simulink model "test_Heaters_Simulink"  (R2016a)
settings: Solver=FixedStepAuto  StartTime=0.0  StopTime=inf  RelTol=1e-3
libraries: arduinolib x5, simulink x1
settings Model: SimulationMode=external  ExtModeTrigDuration=2  Creator=johnh  LastModifiedBy=johnh
settings OptimizationCC: OptimizeModelRefInitCode=on  LifeSpan=1  MaxStackSize=64
settings HardwareCC: ProdBitPerInt=16  ProdBitPerPointer=16  ProdLargestAtomicFloat=None  ProdWordSize=8  ProdHWDeviceType=Atmel->AVR  UseEmbeddedCoderFeatures=off  UseSimulinkCoderFeatures=off
settings RTWCC: SystemTargetFile=ert.tlc  HardwareBoard=Arduino Uno  TemplateMakefile=ert_default_tmf  GenerateReport=on  Toolchain=Arduino AVR v1.6.1  BuildConfiguration=Faster Runs  IncludeHyperlinkInReport=on  LaunchReport=on  GenerateTraceInfo=on  GenerateTraceReport=on  GenerateTraceReportSl=on  GenerateTraceReportSf=on  GenerateTraceReportEml=on
settings CodeAppCC: ForceParamTrailComments=on  IgnoreCustomStorageClasses=off  OperatorAnnotations=on  SimulinkDataObjDesc=on  SFDataObjDesc=on  MATLABFcnDesc=on  InsertBlockDesc=on  MATLABSourceComments=on
settings ERTTargetCC: SupportContinuousTime=on  SupportNonInlinedSFcns=on  SupportVariableSizeSignals=on

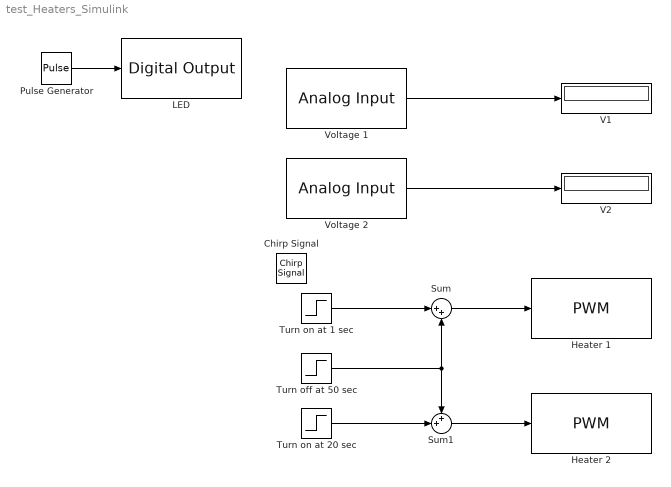
== system test_Heaters_Simulink ==
  Heater 1 : arduinolib/PWM  pinNumber=3  blockPlatform=arduino
  Heater 2 : arduinolib/PWM  pinNumber=5  blockPlatform=arduino
  LED : arduinolib/Digital Output  pinNumber=9  blockPlatform=arduino
  Pulse Generator : DiscretePulseGenerator  Period=10  PulseWidth=5  SampleTime=0.1
  Sum : Sum  Inputs=|++
  Sum1 : Sum  Inputs=++|
  Turn off at 50 sec : Step  Time=50  After=-100  SampleTime=0.1
  Turn on at 1 sec : Step  After=100  SampleTime=0.1
  Turn on at 20 sec : Step  Time=20  After=100  SampleTime=0.1
  V1 : Display
      settings: Decimation=3
  V2 : Display
      settings: Decimation=3
  Voltage 1 : arduinolib/Analog Input  pinNumber=0  sampleTime=0.1  blockPlatform=arduino
  Voltage 2 : arduinolib/Analog Input  pinNumber=2  sampleTime=0.1  blockPlatform=arduino
  Chirp Signal : simulink/Sources/Chirp Signal  IOType=siggen  f1=0.1  T=100  f2=1
  wires:
  Voltage 1/1 -> V1/1
  Turn on at 1 sec/1 -> Sum/1
  Turn off at 50 sec/1 -> Sum/2, Sum1/1
  Sum/1 -> Heater 1/1
  Sum1/1 -> Heater 2/1
  Turn on at 20 sec/1 -> Sum1/2
  Voltage 2/1 -> V2/1
  Pulse Generator/1 -> LED/1
